simulink model "velo_verify"  (R2015a)
settings: Solver=ode3  StartTime=0.0  StopTime=20.0  FixedStep=ts  RelTol=1e-3
values from neighbouring files (symbols this model uses):
  K = 1.904071    [verify_parameter.m]
  T = 0.166667    [verify_parameter.m]
  ts = 1/30    (= 0.0333333333333)    [verify_parameter.m]
  u_offset = 1.5    [verify_parameter.m]
libraries: arduinolib x2
settings Model: SimulationMode=external  ExtModeTrigDuration=2  Creator=shohei  LastModifiedBy=shohei
settings OptimizationCC: OptimizeModelRefInitCode=on  LifeSpan=1
settings DebuggingCC: UnderspecifiedInitializationDetection=Classic  MergeDetectMultiDrivingBlocksExec=none
settings HardwareCC: ProdBitPerInt=16  ProdBitPerPointer=8  ProdIntDivRoundTo=Zero  ProdEndianess=LittleEndian  ProdWordSize=8  ProdHWDeviceType=Atmel->AVR
settings RTWCC: SystemTargetFile=realtime.tlc  GenerateMakefile=off  TemplateMakefile=realtime.tmf  Description=Run on Target Hardware  RTWVerbose=off
settings ERTTargetCC: CombineOutputUpdateFcns=off  ExtModeTransport=3  ExtModeMexFile=ext_serial_win32_comm_rtt  ExtModeMexArgs=0 1 9600  ERTSrcFileBannerTemplate=realtime_code_template.cgt  ERTHdrFileBannerTemplate=realtime_code_template.cgt  ERTDataSrcFileTemplate=realtime_code_template.cgt  ERTDataHdrFileTemplate=realtime_code_template.cgt  ERTCustomFileTemplate=realtime_file_process.tlc

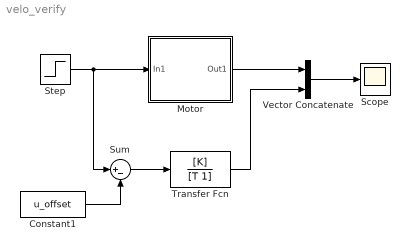
== system velo_verify ==
  Constant1 : Constant  Value=u_offset
  "Motor " : Subsystem
  Scope : Scope
  Step : Step  Time=10  Before=1.5  After=3  SampleTime=ts
  Sum : Sum  Inputs=|+-
  Transfer Fcn : TransferFcn  Numerator=[K]  Denominator=[T 1]
  Vector Concatenate : Concatenate
  wires:
  Step/1 -> Sum/1, "Motor "/1(In1)
  Sum/1 -> Transfer Fcn/1
  Constant1/1 -> Sum/2
  "Motor "/1(Out1) -> Vector Concatenate/1
  Transfer Fcn/1 -> Vector Concatenate/2
  Vector Concatenate/1 -> Scope/1

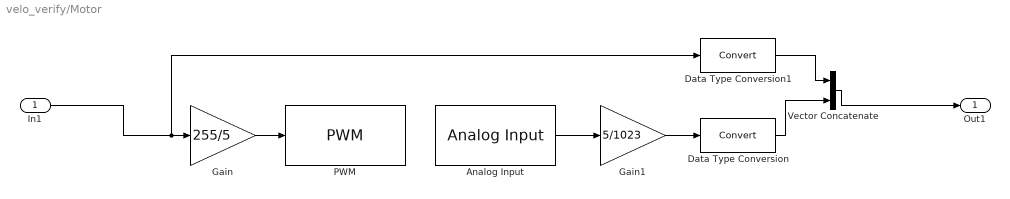
== system velo_verify/Motor  ==
  In1 : Inport
  Analog Input : arduinolib/Analog Input  pinNumber=5  sampleTime=ts  blockPlatform=arduino
  Data Type Conversion : DataTypeConversion
  Data Type Conversion1 : DataTypeConversion
  Gain : Gain  Gain=255/5
  Gain1 : Gain  Gain=5/1023
  PWM : arduinolib/PWM  pinNumber=9  blockPlatform=arduino
  Vector Concatenate : Concatenate
  Out1 : Outport
  wires:
  Data Type Conversion/1 -> Vector Concatenate/2
  Gain1/1 -> Data Type Conversion/1
  Gain/1 -> PWM/1
  Analog Input/1 -> Gain1/1
  Data Type Conversion1/1 -> Vector Concatenate/1
  In1/1 -> Data Type Conversion1/1, Gain/1
  Vector Concatenate/1 -> Out1/1
